simulink model "omni_shooter_model_final"  (R2024b)
settings: Solver=FixedStepDiscrete  StartTime=0.0  StopTime=inf  FixedStep=0.05  RelTol=1e-3
settings Model: Creator=Dell  LastModifiedBy=Dell

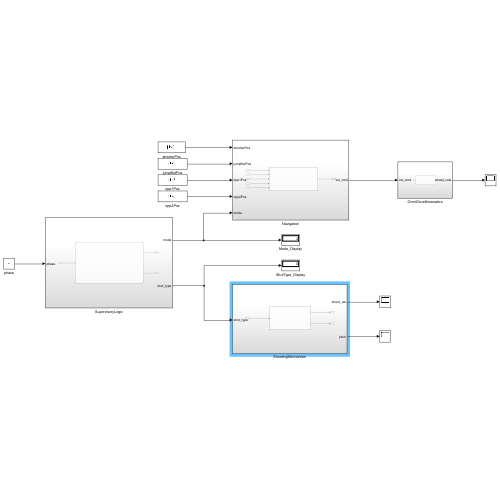
[thumbnail: Simulink's stored preview of the top-level diagram]
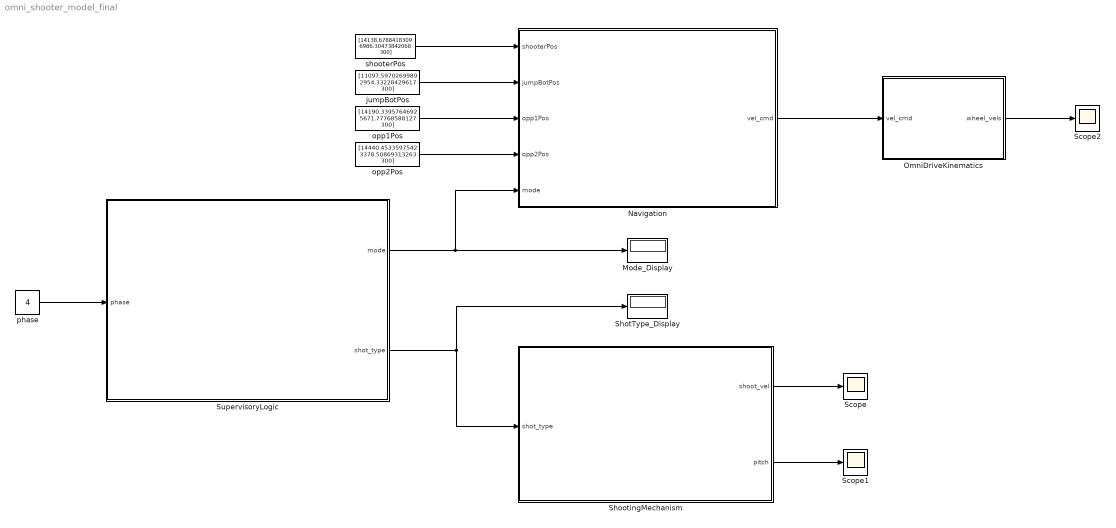
== system omni_shooter_model_final ==
  Mode_Display : Display
  Navigation : Subsystem
  OmniDriveKinematics : Subsystem
  Scope : Scope
  Scope1 : Scope
  Scope2 : Scope
  ShootingMechanism : Subsystem
  ShotType_Display : Display
  SupervisoryLogic : Subsystem
  jumpBotPos : Constant  Value=[11097.5970269989 2954.33228429617 300]
  opp1Pos : Constant  Value=[14190.3395764692 5671.77768588127 300]
  opp2Pos : Constant  Value=[14440.4533597542 3378.50869313263 300]
  phase : Constant  Value=4
  shooterPos : Constant  Value=[14138.6788418309 6986.30473842068 300]
  wires:
  Navigation/1(vel_cmd) -> OmniDriveKinematics/1(vel_cmd)
  SupervisoryLogic/1(mode) -> Mode_Display/1, Navigation/5(mode)
  SupervisoryLogic/2(shot_type) -> ShotType_Display/1, ShootingMechanism/1(shot_type)
  shooterPos/1 -> Navigation/1(shooterPos)
  jumpBotPos/1 -> Navigation/2(jumpBotPos)
  opp1Pos/1 -> Navigation/3(opp1Pos)
  opp2Pos/1 -> Navigation/4(opp2Pos)
  OmniDriveKinematics/1(wheel_vels) -> Scope2/1
  ShootingMechanism/1(shoot_vel) -> Scope/1
  ShootingMechanism/2(pitch) -> Scope1/1
  phase/1 -> SupervisoryLogic/1(phase)

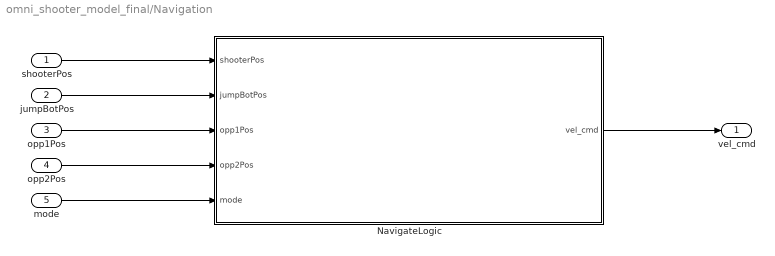
== system omni_shooter_model_final/Navigation ==
  shooterPos : Inport
  jumpBotPos : Inport  Port=2
  opp1Pos : Inport  Port=3
  opp2Pos : Inport  Port=4
  mode : Inport  Port=5
  NavigateLogic : MATLAB Function  TreatAsAtomicUnit=on
  vel_cmd : Outport
  wires:
  shooterPos/1 -> NavigateLogic/1(shooterPos)
  jumpBotPos/1 -> NavigateLogic/2(jumpBotPos)
  opp1Pos/1 -> NavigateLogic/3(opp1Pos)
  opp2Pos/1 -> NavigateLogic/4(opp2Pos)
  mode/1 -> NavigateLogic/5(mode)
  NavigateLogic/1(vel_cmd) -> vel_cmd/1

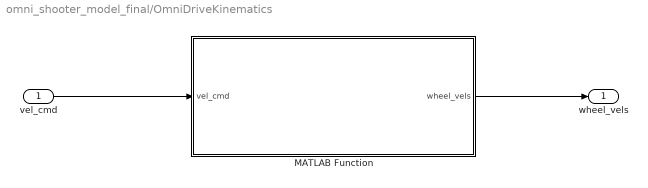
== system omni_shooter_model_final/OmniDriveKinematics ==
  vel_cmd : Inport
  MATLAB Function : MATLAB Function  TreatAsAtomicUnit=on
  wheel_vels : Outport
  wires:
  vel_cmd/1 -> MATLAB Function/1(vel_cmd)
  MATLAB Function/1(wheel_vels) -> wheel_vels/1

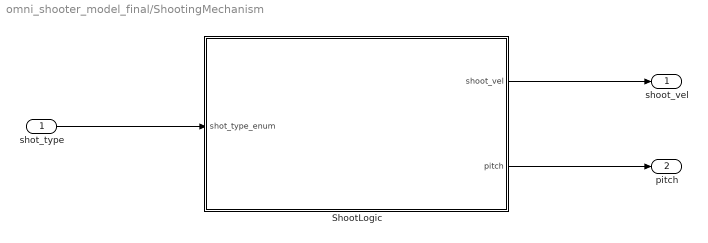
== system omni_shooter_model_final/ShootingMechanism ==
  shot_type : Inport
  ShootLogic : MATLAB Function  TreatAsAtomicUnit=on
  shoot_vel : Outport
  pitch : Outport  Port=2
  wires:
  shot_type/1 -> ShootLogic/1(shot_type_enum)
  ShootLogic/1(shoot_vel) -> shoot_vel/1
  ShootLogic/2(pitch) -> pitch/1

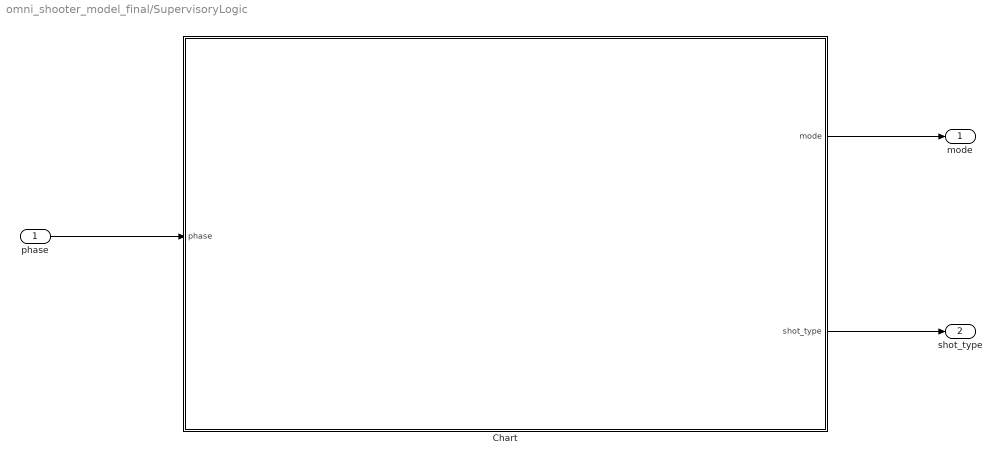
== system omni_shooter_model_final/SupervisoryLogic ==
  phase : Inport
  Chart : Stateflow chart  TreatAsAtomicUnit=on
  mode : Outport
  shot_type : Outport  Port=2
  wires:
  Chart/1(mode) -> mode/1
  Chart/2(shot_type) -> shot_type/1
  phase/1 -> Chart/1(phase)

== matlab function omni_shooter_model_final/ShootingMechanism/ShootLogic ==
  data: shot_type_enum input; shoot_vel output; pitch output
function [shoot_vel, pitch] = ShootLogic(shot_type_enum)
%#codegen
% Shooting logic based on robocon gameplay
% shot_type_enum: 0=no shot, 1=arc shot

% Default outputs
shoot_vel = 0;
pitch = 0;

% Shooting parameters based on shot type
switch shot_type_enum
    case 1 % "arc" shot
        shoot_vel = 4000;
        pitch = 45;
    otherwise % no shot
        shoot_vel = 0;
        pitch = 0;
end
end

== matlab function omni_shooter_model_final/Navigation/NavigateLogic ==
  data: shooterPos input; vel_cmd output; jumpBotPos input; opp1Pos input; opp2Pos input; mode input
function vel_cmd = NavigateLogic(shooterPos, jumpBotPos, opp1Pos, opp2Pos, mode)
%#codegen
% Navigation logic - inputs come from Inport blocks

vel_cmd = zeros(2,1);

% Constants
halfLineX = 7500;
centerY = 4500;
linearSpeed = 400;

% Handle different input sizes safely
if length(shooterPos) >= 2
    shooter_x = shooterPos(1);
    shooter_y = shooterPos(2);
else
    shooter_x = 3000; % default
    shooter_y = 4500; % default
end

% Mode-based navigation (using numeric modes)
switch mode
    case 2 % toHalfCourt
        target_x = halfLineX - 1000;
        target_y = centerY;
        dx = target_x - shooter_x;
        dy = target_y - shooter_y;
        distance = sqrt(dx*dx + dy*dy);
        if distance > 0
            vel_cmd(1) = (dx / distance) * linearSpeed;
            vel_cmd(2) = (dy / distance) * linearSpeed;
        end
        
    case 3 % navigateToArc
        arcCenter_x = 14400;
        arcCenter_y = 4500;
        arcRadius = 2500;
        target_x = arcCenter_x + arcRadius * cos(pi);
        target_y = arcCenter_y + arcRadius * sin(pi);
        dx = target_x - shooter_x;
        dy = target_y - shooter_y;
        distance = sqrt(dx*dx + dy*dy);
        if distance > 0
            vel_cmd(1) = (dx / distance) * linearSpeed;
            vel_cmd(2) = (dy / distance) * linearSpeed;
        end
        
    case 4 % aroundArc
        arcCenter_x = 14400;
        arcCenter_y = 4500;
        currentAngle = atan2(shooter_y - arcCenter_y, shooter_x - arcCenter_x);
        vel_cmd(1) = -sin(currentAngle) * linearSpeed * 0.5;
        vel_cmd(2) = cos(currentAngle) * linearSpeed * 0.5;
end
end

== stateflow chart omni_shooter_model_final/SupervisoryLogic/Chart ==
  state IDLE
    entry:
    mode = 1;
    shot_type = 0;
  state TO_HALF_COURT
    entry:
    mode = 2;
    shot_type = 0;
  state GAME_COMPLETE
    entry:
    mode = 6;
    shot_type = 0;
  state SHOOT
    entry:
    mode = 5;
    shot_type = 1;
  state NAVIGATE_TO_ARC
    entry:
    mode = 3;
    shot_type = 0;
  state AROUND_ARC
    entry:
    mode = 4;
    shot_type = 0;
  (default) -> IDLE
  IDLE -> TO_HALF_COURT : after(1,sec)
  GAME_COMPLETE -> IDLE : after(5,sec)
  SHOOT -> GAME_COMPLETE : after(3,sec)
  TO_HALF_COURT -> NAVIGATE_TO_ARC : [phase == 3]
  AROUND_ARC -> SHOOT : [phase == 5]
  NAVIGATE_TO_ARC -> AROUND_ARC : [phase == 4]
  data: mode output double; shot_type output double; phase input double size=1

== matlab function omni_shooter_model_final/OmniDriveKinematics/MATLAB Function ==
  data: vel_cmd input; wheel_vels output
function wheel_vels = OmniKinematics(vel_cmd)
%#codegen
% Convert velocity commands to wheel velocities for omni-drive

% Robot parameters
wheelRadius = 50; % mm
robotRadius = 200; % mm

% Extract velocity components
if length(vel_cmd) >= 2
    vx = vel_cmd(1);
    vy = vel_cmd(2);
else
    vx = 0;
    vy = 0;
end

omega = 0; % No rotation for now

% Omni-wheel kinematics matrix (4-wheel configuration)
% Wheel arrangement: front-left, front-right, back-right, back-left
wheel_vels = (1/wheelRadius) * [
    -vx + vy + robotRadius * omega;  % Front-left
     vx + vy + robotRadius * omega;  % Front-right  
     vx - vy + robotRadius * omega;  % Back-right
    -vx - vy + robotRadius * omega   % Back-left
];
end
